simulink model "diagram_analog_scalar"  (Simulink 7.5)
settings: Solver=ode4  StartTime=0.0  StopTime=10.0  FixedStep=0.001  RelTol=1e-3
settings Model: Creator=Dell  LastModifiedBy=huiliang

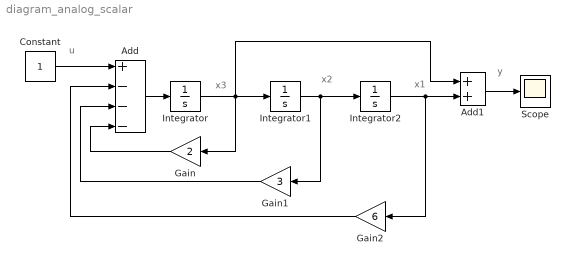
== system diagram_analog_scalar ==
  note: x3
  note: x2
  note: x1
  note: y
  note: u
  Add : Sum  Inputs=+---  OutDataType=fixdt(1, 16)  OutScaling=2^-10
  Add1 : Sum  OutDataType=fixdt(1, 16)  OutScaling=2^-10
  Constant : Constant  OutDataType=fixdt(1, 16)  OutScaling=2^0
  Gain : Gain  Gain=2  ParameterDataType=fixdt(1, 16)  ParameterScaling=2^0  OutDataType=fixdt(1, 16)  OutScaling=2^0
  Gain1 : Gain  Gain=3  ParameterDataType=fixdt(1, 16)  ParameterScaling=2^0  OutDataType=fixdt(1, 16)  OutScaling=2^0
  Gain2 : Gain  Gain=6  ParameterDataType=fixdt(1, 16)  ParameterScaling=2^0  OutDataType=fixdt(1, 16)  OutScaling=2^0
  Integrator : Integrator
  Integrator1 : Integrator
  Integrator2 : Integrator
  Scope : Scope
      settings: TimeRange=10  YMin=-0.2  YMax=0.6000000000000001  MaxDataPoints=10000
  wires:
  Integrator1/1 -> Integrator2/1, Gain1/1
  Integrator/1 -> Integrator1/1, Gain/1, Add1/1
  Add/1 -> Integrator/1
  Integrator2/1 -> Add1/2, Gain2/1
  Gain/1 -> Add/4
  Gain1/1 -> Add/3
  Gain2/1 -> Add/2
  Constant/1 -> Add/1
  Add1/1 -> Scope/1
